simulink model "PNEUMA"  (R2023b)
settings: Solver=ode23tb  StartTime=0  StopTime=3600  FixedStep=0.001  MaxStep=time_step_new  RelTol=0.01  EnableMultiTasking=on
values from neighbouring files (symbols this model uses):
  A = 20.9    [Gas_Exchange_IC.m]    (also in getPneumonia.m = (LF1-LF2)/(1-exp(Rresolve*(t2(end)-t2(1)))))
  a1 = 0.3836    [Dissociation_Spencer_IC.m]    (also in Gas_Exchange_IC.m; Respiratory_IC.m)
  a2 = 1.819    [Dissociation_Spencer_IC.m]    (also in Gas_Exchange_IC.m; Respiratory_IC.m)
  alpha1 = 0.02598    [Dissociation_Spencer_IC.m]    (also in Gas_Exchange_IC.m; Respiratory_IC.m)
  alpha2 = 0.05591    [Dissociation_Spencer_IC.m]    (also in Gas_Exchange_IC.m; Respiratory_IC.m)
  B = 92.8    [Gas_Exchange_IC.m]    (also in getPneumonia.m = LungFunction(end)-A)
  beta1 = 0.012275    [Dissociation_Spencer_IC.m]    (also in Gas_Exchange_IC.m; Respiratory_IC.m)
  beta2 = 0.03255    [Dissociation_Spencer_IC.m]    (also in Gas_Exchange_IC.m; Respiratory_IC.m)
  C = 10570    [Gas_Exchange_IC.m]
  C1 = 9    [Dissociation_Spencer_IC.m]    (also in Gas_Exchange_IC.m; Respiratory_IC.m)
  C2 = 87.00    (= 87)    [Dissociation_Spencer_IC.m]    (also in Gas_Exchange_IC.m; Respiratory_IC.m)
  Circadian_Period = 24    [Respiratory_IC.m]    (also in State_UA_Khoo_IC.m)
  CvCO2IC = 0.5116    [Body_Khoo_IC.m]    (also in Gas_Exchange_IC.m; Respiratory_IC.m = 0.5247)
  CvO2IC = 0.1672    [Body_Khoo_IC.m]    (also in Gas_Exchange_IC.m; Respiratory_IC.m = 0.1639)
  D = -5.251    [Gas_Exchange_IC.m]
  Dead1CO2IC = 0.1020    (= 0.102)    [Dead_Space_Khoo_IC.m]    (also in Gas_Exchange_IC.m; Respiratory_IC.m = 39.5616)
  Dead1O2IC = 149.8824    [Dead_Space_Khoo_IC.m]    (also in Gas_Exchange_IC.m; Respiratory_IC.m = 104.3637)
  Dead2CO2IC = 0.5274    [Dead_Space_Khoo_IC.m]    (also in Gas_Exchange_IC.m; Respiratory_IC.m = 39.6736)
  Dead2O2IC = 149.3923    [Dead_Space_Khoo_IC.m]    (also in Gas_Exchange_IC.m; Respiratory_IC.m = 104.2258)
  Dead3CO2IC = 2.2996    [Dead_Space_Khoo_IC.m]    (also in Gas_Exchange_IC.m; Respiratory_IC.m = 39.8127)
  Dead3O2IC = 147.3503    [Dead_Space_Khoo_IC.m]    (also in Gas_Exchange_IC.m; Respiratory_IC.m = 104.0505)
  Dead4CO2IC = 8.2293    [Dead_Space_Khoo_IC.m]    (also in Gas_Exchange_IC.m; Respiratory_IC.m = 40.0061)
  Dead4O2IC = 140.5179    [Dead_Space_Khoo_IC.m]    (also in Gas_Exchange_IC.m; Respiratory_IC.m = 103.8005)
  Dead5CO2IC = 22.0757    [Dead_Space_Khoo_IC.m]    (also in Gas_Exchange_IC.m; Respiratory_IC.m = 40.3359)
  Dead5O2IC = 124.5641    [Dead_Space_Khoo_IC.m]    (also in Gas_Exchange_IC.m; Respiratory_IC.m = 103.3579)
  DtotalIC = 0.3    [NeuroMuscular_IC.m]    (also in Respiratory_IC.m = 0.32)
  E_CW = 5    [Pleural_Schuessler_IC.m]    (also in Pmus_Flow_Younes_IC.m; Resp_Mech_IC.m; Respiratory_IC.m)
  E_L = 5    [Pleural_Schuessler_IC.m]    (also in Pmus_Flow_Younes_IC.m; Resp_Mech_IC.m; Respiratory_IC.m)
  fc = 0.4/60    (= 0.00666666666667)    [Respiratory_IC.m]    (also in State_UA_Khoo_IC.m)
  fcs_max = 47.78    [Cardiovascular_IC.m]    (also in Reflex_Ursino_IC.m)
  fcs_min = 2.52    [Cardiovascular_IC.m]    (also in Reflex_Ursino_IC.m)
  fcs_zero = 25    [Respiratory_IC.m]
  FlowIC = 0    [Pmus_Flow_Younes_IC.m]    (also in Resp_Mech_IC.m; Respiratory_IC.m)
  fp_inf = 6.3    [Respiratory_IC.m]
  fp_zero = 3.2    [Respiratory_IC.m]
  fs_inf = 2.10    (= 2.1)    [Respiratory_IC.m]
  fs_zero = 16.11    [Respiratory_IC.m]
  ftbs_min = 0.1    [Cardiovascular_IC.m]    (also in SA_Node_Ursino_IC.m)
  gc = 0.008/60    (= 0.000133333333333)    [Respiratory_IC.m]    (also in State_UA_Khoo_IC.m)
  h = 0.0183    [Brain_Khoo_IC.m]    (also in Gas_Exchange_IC.m; Respiratory_IC.m)
  HP_basal = 0.58    [Cardiovascular_IC.m]    (also in SA_Node_Ursino_IC.m)
  Ic = 45    [Gas_Exchange_IC.m]    (also in Respiratory_IC.m; Vent_Drive_Khoo_IC.m)
  IpCO2 = 38    [Gas_Exchange_IC.m]    (also in Respiratory_IC.m; Vent_Drive_Khoo_IC.m)
  IpO2 = 102.4    [Gas_Exchange_IC.m]    (also in Respiratory_IC.m; Vent_Drive_Khoo_IC.m)
  K1 = 13    [Dissociation_Spencer_IC.m]    (also in Gas_Exchange_IC.m; Respiratory_IC.m)
  K2 = 194.4    [Dissociation_Spencer_IC.m]    (also in Gas_Exchange_IC.m; Respiratory_IC.m)
  k_cs = 11.758    [Cardiovascular_IC.m]    (also in Reflex_Ursino_IC.m)
  k_p = 7.06    [Respiratory_IC.m]
  k_s = 0.07    [Respiratory_IC.m]
  lambda = 863    [Gas_Exchange_IC.m]    (also in Lungs_Khoo_IC.m; Respiratory_IC.m)
  Mech_Vent_pressure = 17    [Mech_vent_test.m]
  MRbCO2 = 0.0517    [Brain_Khoo_IC.m]    (also in Gas_Exchange_IC.m; Respiratory_IC.m)
  MRCO2 = 0.0033    [Body_Khoo_IC.m]    (also in Gas_Exchange_IC.m; Respiratory_IC.m)
  MRO2 = 0.0038    [Body_Khoo_IC.m]    (also in Gas_Exchange_IC.m; Respiratory_IC.m)
  NM_block_gain = 1    [Mech_vent_test.m]
  PACO2_delayIC = 39.6041    [Cardio_Mix_Lange_IC.m]    (also in Gas_Exchange_IC.m; Respiratory_IC.m = 40.4448)
  PaCO2firstIC = 0.2150    (= 0.215)    [Cardio_Mix_Lange_IC.m]    (also in Gas_Exchange_IC.m; Respiratory_IC.m = -0.2465)
  PACO2IC = 37.1484    [Gas_Exchange_IC.m]    (also in Lungs_Khoo_IC.m; Respiratory_IC.m = 40.9432)
  PaCO2secondIC = 38.4577    [Cardio_Mix_Lange_IC.m]    (also in Gas_Exchange_IC.m; Respiratory_IC.m = 40.3928)
  PAO2_delayIC = 103.8436    [Cardio_Mix_Lange_IC.m]    (also in Gas_Exchange_IC.m; Respiratory_IC.m = 103.1223)
  PaO2firstIC = -0.2838    [Cardio_Mix_Lange_IC.m]    (also in Gas_Exchange_IC.m; Respiratory_IC.m = 0.3557)
  PAO2IC = 107.1983    [Gas_Exchange_IC.m]    (also in Lungs_Khoo_IC.m; Respiratory_IC.m = 102.5153)
  PaO2secondIC = 105.4828    [Cardio_Mix_Lange_IC.m]    (also in Gas_Exchange_IC.m; Respiratory_IC.m = 103.1435)
  PbCO2IC = 48.2858    [Brain_Khoo_IC.m]    (also in Gas_Exchange_IC.m; Respiratory_IC.m = 48.5383)
  PICO2 = 0    [Dead_Space_Khoo_IC.m]    (also in Gas_Exchange_IC.m; Respiratory_IC.m)
  PIO2 = 150    [Dead_Space_Khoo_IC.m]    (also in Gas_Exchange_IC.m; Respiratory_IC.m)
  PIO2_change = -90    [Mech_vent_test.m]    (also in Respiratory_IC.m = 0)
  Pn = 90    [Cardiovascular_IC.m]    (also in Reflex_Ursino_IC.m)
  Pt_frcIC1 = 0    [Pmus_Flow_Younes_IC.m]    (also in Resp_Mech_IC.m; Respiratory_IC.m)
  Pt_frcIC2 = 0    [Pmus_Flow_Younes_IC.m]    (also in Resp_Mech_IC.m; Respiratory_IC.m)
  QdBo = 0.8333    [Brain_Khoo_IC.m]    (also in Gas_Exchange_IC.m; Respiratory_IC.m)
  R_AW = 1.27    [Pleural_Schuessler_IC.m]    (also in Pmus_Flow_Younes_IC.m; Resp_Mech_IC.m; Respiratory_IC.m)
  R_CW = 1.03    [Pleural_Schuessler_IC.m]    (also in Pmus_Flow_Younes_IC.m; Resp_Mech_IC.m; Respiratory_IC.m)
  R_L = 1.69    [Pleural_Schuessler_IC.m]    (also in Pmus_Flow_Younes_IC.m; Resp_Mech_IC.m; Respiratory_IC.m)
  RC = 0.06    [Pleural_Schuessler_IC.m]    (also in Pmus_Flow_Younes_IC.m; Resp_Mech_IC.m; Respiratory_IC.m)
  rc = 0.2/60    (= 0.00333333333333)    [Respiratory_IC.m]    (also in State_UA_Khoo_IC.m)
  SbCO2 = 0.3600    (= 0.36)    [Brain_Khoo_IC.m]    (also in Gas_Exchange_IC.m; Respiratory_IC.m)
  SCO2 = 0.0043    [Brain_Khoo_IC.m]    (also in Gas_Exchange_IC.m; Respiratory_IC.m)
  SWAo = 0.007    [Respiratory_IC.m]    (also in State_UA_Khoo_IC.m)
  T1 = 1    [Cardio_Mix_Lange_IC.m]    (also in Gas_Exchange_IC.m; Respiratory_IC.m)
  T2 = 2    [Cardio_Mix_Lange_IC.m]    (also in Gas_Exchange_IC.m; Respiratory_IC.m)
  t_end_new = 4*24*60*60    (= 345600)    [Mech_vent_test.m]
  t_end_UA = 0    [Respiratory_IC.m]    (also in State_UA_Khoo_IC.m)
  t_Mech_Vent_duration = 0    [Mech_vent_test.m]
  t_Mech_Vent_start = 0    [Mech_vent_test.m]
  t_Mueller_duration = 0    [NeuroMuscular_IC.m]
  t_Mueller_insp = 0    [NeuroMuscular_IC.m]
  t_Mueller_start = 0    [NeuroMuscular_IC.m]
  t_NM_block_duration = 0    [Mech_vent_test.m]
  t_NM_block_start = 0    [Mech_vent_test.m]
  t_O2_duration = 0    [Mech_vent_test.m]    (also in Respiratory_IC.m)
  t_O2_start = 0    [Mech_vent_test.m]    (also in Respiratory_IC.m)
  t_start_new = 0    [Mech_vent_test.m]
  t_start_UA = 0    [Respiratory_IC.m]    (also in State_UA_Khoo_IC.m)
  t_valsalva_duration = 0    [NeuroMuscular_IC.m]
  t_valsalva_insp = 0    [NeuroMuscular_IC.m]
  t_valsalva_start = 0    [NeuroMuscular_IC.m]
  time_step = time_step    [acquire_data.m]    (also in acquire_data_save.m)
  VC = 5    [Pmus_Flow_Younes_IC.m]    (also in Resp_Mech_IC.m; Respiratory_IC.m)
  Vdead1 = 0.03    [Dead_Space_Khoo_IC.m]    (also in Gas_Exchange_IC.m; Respiratory_IC.m)
  Vdead2 = 0.03    [Dead_Space_Khoo_IC.m]    (also in Gas_Exchange_IC.m; Respiratory_IC.m)
  Vdead3 = 0.03    [Dead_Space_Khoo_IC.m]    (also in Gas_Exchange_IC.m; Respiratory_IC.m)
  Vdead4 = 0.03    [Dead_Space_Khoo_IC.m]    (also in Gas_Exchange_IC.m; Respiratory_IC.m)
  Vdead5 = 0.03    [Dead_Space_Khoo_IC.m]    (also in Gas_Exchange_IC.m; Respiratory_IC.m)
  Ventilator_rate = 12    [Mech_vent_test.m]
  VTCO2 = 15    [Body_Khoo_IC.m]    (also in Gas_Exchange_IC.m; Respiratory_IC.m)
  VtIC = 0    [Pmus_Flow_Younes_IC.m]    (also in Resp_Mech_IC.m; Respiratory_IC.m)
  VTO2 = 6    [Body_Khoo_IC.m]    (also in Gas_Exchange_IC.m; Respiratory_IC.m)
  Z = 0.0227    [Dissociation_Spencer_IC.m]    (also in Gas_Exchange_IC.m; Respiratory_IC.m)
undefined symbols (not defined in the file or in its folder): A_0_ua, alpha_E_FFA_Heart, alpha_E_FFA_muscle, alpha_E_GLC_Heart, alpha_E_GLC_muscle, alpha_E_GLY_muscle, alpha_E_PYR_muscle, alpha_E_TGL_adipose, alpha_E_TGL_GI, alpha_E_TGL_Heart, alpha_E_TGL_muscle, Arousal_UAIC, C_ua_awake, Cbp, Cbv, Ce_0, Cep, Cev, Chp, Chv, Cla, Clamp_class, Cmp, Cmv, Cpa, CPAP_pressure, Cpp, Cpv, Cra, Csa, Csp, Csv, CvbO2_n, CvhO2_n, CvmO2_n, DAY, delay, DietBlock, Dx, Fb, fchemo_max, fchemo_min, fchemoIC, flsIC, Ftas_I0, ftas_min, ftas_r0, FVC_activation, gain_E, Gamma, Gas_sleep, Gas_sleepM, Gb, Gblock, GbO2, Gbs_sleep, gcc_sa, gcc_sb, gcc_sp, Gclamp ... (+144)
libraries: simulink x4, dspstat3 x4, simulink_extras x2
(part 6 of 8)

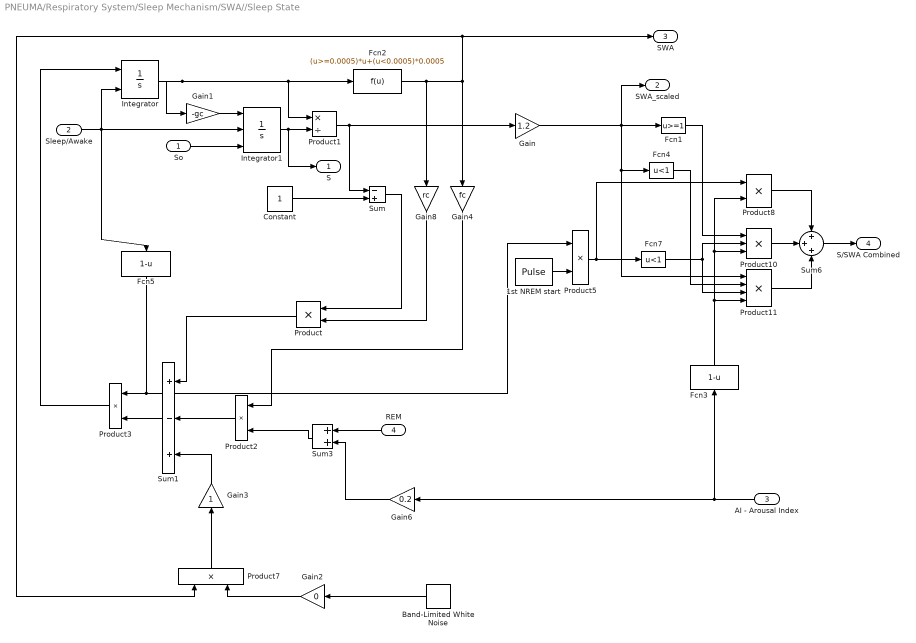
== system PNEUMA/Respiratory System/Sleep Mechanism/SWA//Sleep State ==
  So : Inport
  Sleep/Awake : Inport  Port=2
  AI - Arousal Index : Inport  Port=3
  REM : Inport  Port=4
  1st NREM start : DiscretePulseGenerator  PulseType=Time based  Period=Circadian_Period*3600  PulseWidth=100 - 85 *1.8 /Circadian_Period  PhaseDelay=3600*1.8*0.85+5
  Band-Limited White Noise : simulink/Sources/Band-Limited White Noise  Cov=[0.1]  Ts=0.1  seed=[23341]
  Constant : Constant
  Fcn1 : Fcn  Expr=u>=1
  Fcn2 : Fcn  Expr=(u>=0.0005)*u+(u<0.0005)*0.0005
  Fcn3 : Fcn  Expr=1-u
  Fcn4 : Fcn  Expr=u<1
  Fcn5 : Fcn  Expr=1-u
  Fcn7 : Fcn  Expr=u<1
  Gain : Gain  Gain=1.2
  Gain1 : Gain  Gain=-gc  SaturateOnIntegerOverflow=on  OutDataTypeStr=Inherit: Same as input  ParamDataTypeStr=Inherit: Same as input
  Gain2 : Gain  Gain=0  SaturateOnIntegerOverflow=on  OutDataTypeStr=Inherit: Same as input  ParamDataTypeStr=Inherit: Same as input
  Gain3 : Gain  SaturateOnIntegerOverflow=on  OutDataTypeStr=Inherit: Same as input  ParamDataTypeStr=Inherit: Same as input
  Gain4 : Gain  Gain=fc  SaturateOnIntegerOverflow=on  OutDataTypeStr=Inherit: Same as input  ParamDataTypeStr=Inherit: Same as input
  Gain6 : Gain  Gain=0.2  SaturateOnIntegerOverflow=on  OutDataTypeStr=Inherit: Same as input  ParamDataTypeStr=Inherit: Same as input
  Gain8 : Gain  Gain=rc  SaturateOnIntegerOverflow=on  OutDataTypeStr=Inherit: Same as input  ParamDataTypeStr=Inherit: Same as input
  Integrator : Integrator  ExternalReset=either  InitialCondition=SWAo  LimitOutput=on  UpperSaturationLimit=1  LowerSaturationLimit=0
  Integrator1 : Integrator  ExternalReset=falling  InitialConditionSource=external  InitialCondition=0.8  LimitOutput=on
  Product{,2..3,7..8} (5 alike) : Product  InputSameDT=on  SaturateOnIntegerOverflow=on  OutDataTypeStr=Inherit: Same as first input
  Product1 : Product  Inputs=*/  InputSameDT=on  SaturateOnIntegerOverflow=on  OutDataTypeStr=Inherit: Same as first input
  Product10 : Product  Inputs=3  InputSameDT=on  SaturateOnIntegerOverflow=on  OutDataTypeStr=Inherit: Same as first input
  Product11 : Product  Inputs=4  InputSameDT=on  SaturateOnIntegerOverflow=on  OutDataTypeStr=Inherit: Same as first input
  Product5 : Product  Inputs=**  InputSameDT=on  SaturateOnIntegerOverflow=on  OutDataTypeStr=Inherit: Same as first input
  Sum : Sum  Inputs=-+  InputSameDT=on  SaturateOnIntegerOverflow=on  OutDataTypeStr=Inherit: Same as first input
  Sum1 : Sum  Inputs=+-+  InputSameDT=on  SaturateOnIntegerOverflow=on  OutDataTypeStr=Inherit: Same as first input
  Sum3 : Sum  InputSameDT=on  SaturateOnIntegerOverflow=on  OutDataTypeStr=Inherit: Same as first input
  Sum6 : Sum  Inputs=+++  InputSameDT=on  SaturateOnIntegerOverflow=on  OutDataTypeStr=Inherit: Same as first input
  S : Outport
  SWA_scaled : Outport  Port=2
  SWA : Outport  Port=3
  S/SWA Combined : Outport  Port=4
  wires:
  Fcn4/1 -> Product11/2
  Fcn7/1 -> Product11/3, Product10/2
  Product10/1 -> Sum6/2
  Product11/1 -> Sum6/3
  Sum6/1 -> S/SWA Combined/1
  Product8/1 -> Sum6/1
  Gain2/1 -> Product7/2
  Product7/1 -> Gain3/1
  Gain6/1 -> Sum3/2
  AI - Arousal Index/1 -> Gain6/1, Fcn3/1
  Sum3/1 -> Product2/2
  Constant/1 -> Sum/2
  Product1/1 -> Sum/1, Gain/1
  Gain1/1 -> Integrator1/1
  Integrator/1 -> Product1/1, Fcn2/1, Gain1/1
  Sum/1 -> Product/1
  Product/1 -> Sum1/1
  Product2/1 -> Sum1/2
  Gain3/1 -> Sum1/3
  Integrator1/1 -> Product1/2, S/1
  Sleep/Awake/1 -> Integrator1/2, Fcn5/1, Integrator/2
  So/1 -> Integrator1/3
  Fcn2/1 -> Gain4/1, Product7/1, SWA/1, Gain8/1
  Gain/1 -> SWA_scaled/1, Fcn1/1, Product11/1, Fcn4/1
  Gain4/1 -> Product2/1
  Gain8/1 -> Product/2
  Sum1/1 -> Product3/2
  Product3/1 -> Integrator/1
  Fcn5/1 -> Product3/1, Product5/1
  Fcn3/1 -> Product8/2, Product10/3, Product11/4
  Band-Limited White Noise/1 -> Gain2/1
  Product5/1 -> Fcn7/1, Product8/1
  1st NREM start/1 -> Product5/2
  Fcn1/1 -> Product10/1
  REM/1 -> Sum3/1

== system PNEUMA/Respiratory System/Sleep Mechanism/Saving CircadianProcess ==
  In1 : Inport
  Clock : Clock
  Gain : Gain  Gain=1/(3600*24*DAY)
  Rounding Function : Rounding
  Switch Case : SwitchCase  CaseConditions={0,1,2,3,4,5,6,7,8}  SampleTime=sampletime
  Switch Case Action Subsystem : Subsystem  TreatAsAtomicUnit=on
  Switch Case Action Subsystem1 : Subsystem  TreatAsAtomicUnit=on
  Switch Case Action Subsystem2 : Subsystem  TreatAsAtomicUnit=on
  Switch Case Action Subsystem3 : Subsystem  TreatAsAtomicUnit=on
  Switch Case Action Subsystem4 : Subsystem  TreatAsAtomicUnit=on
  Switch Case Action Subsystem5 : Subsystem  TreatAsAtomicUnit=on
  Switch Case Action Subsystem6 : Subsystem  TreatAsAtomicUnit=on
  Switch Case Action Subsystem7 : Subsystem  TreatAsAtomicUnit=on
  Switch Case Action Subsystem8 : Subsystem  TreatAsAtomicUnit=on
  Switch Case Action Subsystem9 : Subsystem  TreatAsAtomicUnit=on
  wires:
  Clock/1 -> Gain/1
  Switch Case/1 -> Switch Case Action Subsystem/Action
  Switch Case/2 -> Switch Case Action Subsystem1/Action
  Switch Case/3 -> Switch Case Action Subsystem2/Action
  Switch Case/10 -> Switch Case Action Subsystem3/Action
  Rounding Function/1 -> Switch Case/1
  In1/1 -> Switch Case Action Subsystem/1(In1), Switch Case Action Subsystem1/1(In1), Switch Case Action Subsystem2/1(In1), Switch Case Action Subsystem5/1(In1), Switch Case Action Subsystem3/1(In1), Switch Case Action Subsystem9/1(In1), Switch Case Action Subsystem8/1(In1), Switch Case Action Subsystem7/1(In1), Switch Case Action Subsystem6/1(In1), Switch Case Action Subsystem4/1(In1)
  Gain/1 -> Rounding Function/1
  Switch Case/4 -> Switch Case Action Subsystem4/Action
  Switch Case/5 -> Switch Case Action Subsystem5/Action
  Switch Case/6 -> Switch Case Action Subsystem6/Action
  Switch Case/7 -> Switch Case Action Subsystem7/Action
  Switch Case/8 -> Switch Case Action Subsystem8/Action
  Switch Case/9 -> Switch Case Action Subsystem9/Action

== system PNEUMA/Respiratory System/Sleep Mechanism/Triggered Subsystem ==
  In1 : Inport
  Trigger : TriggerPort  VariantControl=(inherit)
  Out1 : Outport
  wires:
  In1/1 -> Out1/1

== system PNEUMA/Respiratory System/Upper_Airway_Mechanism/State-dependent Upper Airway model ==
  SI Sleep Wake State Index : Inport
  AI - Arousal Index : Inport  Port=2
  External Pressure : Inport  Port=3
  Sleep/Awake : Inport  Port=4
  SWA/S : Inport  Port=5
  Airway Cond Saturation2 : Saturate  UpperLimit=1  LowerLimit=0
  Fcn1 : Fcn  Expr="((u(1) >=1.0) * u(2) * (1 + 0.3 * (1 - u(3)) * (1-u(4)) )  + ( u(1)<1.0) * u(1) * u(2) ) *(1- u(5))* u(1)"
  Integrator : Integrator  ExternalReset=rising  InitialCondition=Arousal_UAIC
  Mux1 : Mux  Inputs=5
  PE gain2 : Gain  Gain=1/15  SaturateOnIntegerOverflow=on  OutDataTypeStr=Inherit: Same as input  ParamDataTypeStr=Inherit: Same as input
  S_UA : Constant  Value=0.05
  sum3 : Sum  Inputs=-+  InputSameDT=on  SaturateOnIntegerOverflow=on  OutDataTypeStr=Inherit: Same as first input
  tag scope: Arousal_UAIC=global
  wires:
  AI - Arousal Index/1 -> Integrator/2, Mux1/5
  SI Sleep Wake State Index/1 -> Mux1/1
  SWA/S/1 -> Mux1/3
  Sleep/Awake/1 -> Mux1/4
  S_UA/1 -> sum3/2
  sum3/1 -> Airway Cond Saturation2/1
  External Pressure/1 -> PE gain2/1
  PE gain2/1 -> sum3/1
  Mux1/1 -> Fcn1/1
  Airway Cond Saturation2/1 -> Mux1/2
  Fcn1/1 -> Integrator/1
  Integrator/1 -> [Arousal_UAIC]

== system PNEUMA/Respiratory System/Upper_Airway_Mechanism/Upper_Airway_Model ==
  SI Sleep Wake State Index : Inport
  Respiratory Rhythm : Inport  Port=2
  Q_total Total Respiratory Flow Airways : Inport  Port=3
  Pleural Pressure : Inport  Port=4
  Tidal Volume : Inport  Port=5
  Total Ventilatory Drive : Inport  Port=6
  Sleep/awake : Inport  Port=7
  Enable : EnablePort
  " Flow in Upper Airway" : Subsystem
  " Pressure in Upper Airway" : Subsystem
  Coefficient1 : Gain  SaturateOnIntegerOverflow=on  OutDataTypeStr=Inherit: Same as input  ParamDataTypeStr=Inherit: Same as input
  Mux : Mux  Inputs=2
  Sum2 : Sum  SaturateOnIntegerOverflow=on
  Upper Airway Conductance3 : Subsystem
  Upper Airway Scope : Scope  NumInputPorts=12
  Upper_Airway_Compliance : Subsystem
  "Y_ua Upper Airway Conductance " : Outport  InitialOutput=[0]
  wires:
  Q_total Total Respiratory Flow Airways/1 -> Upper Airway Scope/8, Coefficient1/1  "Q_total"
  SI Sleep Wake State Index/1 -> Upper_Airway_Compliance/1("SI Sleep Wake State Index "), Upper Airway Scope/1  "SI Sleep Wake State Index"
  Pleural Pressure/1 -> Upper Airway Scope/4, " Pressure in Upper Airway"/1(P_pl Pleural Pressure)  "P_pl Pleural Pressure"
  Sum2/1 -> " Pressure in Upper Airway"/2(Q_la Lower Airway Flow), Upper Airway Scope/10  "Q_la Lower Airway Flow"
  " Pressure in Upper Airway"/1("P_ua Upper Airway Pressure ") -> " Flow in Upper Airway"/2(P_ua Pressure in Upper Airways), Upper Airway Conductance3/2(P_ua_Upper Airway Pressure), Mux/2, Upper Airway Scope/5  "P_ua"
  Upper Airway Conductance3/2(P_crit) -> Mux/1  "P_crit"
  Upper_Airway_Compliance/1(C_ua Upper Airway Compliance) -> " Flow in Upper Airway"/1(C_ua Upper Airway Compliance), Upper Airway Conductance3/1(C_ua_Upper_Airway_Compliance), Upper Airway Scope/11  "C_ua Upper Airway Copmliance"
  " Flow in Upper Airway"/1("Q_ua Upper Airway Flow ") -> Upper Airway Scope/9, Sum2/1  "Q_ua Upper Airway Flow"
  Upper Airway Conductance3/1(Y_ua_Upper Airway Conductance) -> Upper Airway Scope/12, "Y_ua Upper Airway Conductance "/1  "Y_ua Upper Airway Conductance"
  Total Ventilatory Drive/1 -> Upper Airway Scope/2  "Ventilatory Drive"
  Mux/1 -> Upper Airway Scope/6  "P_ua vs. P_cirt"
  Tidal Volume/1 -> Upper Airway Scope/7  "Tidal Volume"
  Respiratory Rhythm/1 -> Upper Airway Scope/3  "Respiratory Rhythm"
  Sleep/awake/1 -> Upper_Airway_Compliance/2(Sleep/awake)
  Coefficient1/1 -> Sum2/2

== system PNEUMA/Ventilator/Saving CONTROLLER/Switch Case Action Subsystem ==
  In1 : Inport
  Action Port : ActionPort  ActionPortLabel=case [ 0 ]:
  To File : ToFile  Filename=CONTROLLER1.mat  MatrixName=CONTROLLER  SampleTime=sampletime
  wires:
  In1/1 -> To File/1

== system PNEUMA/Ventilator/Saving CONTROLLER/Switch Case Action Subsystem1 ==
  In1 : Inport
  Action Port : ActionPort  ActionPortLabel=case [ 1 ]:
  To File : ToFile  Filename=CONTROLLER2.mat  MatrixName=CONTROLLER  SampleTime=sampletime
  wires:
  In1/1 -> To File/1

== system PNEUMA/Ventilator/Saving CONTROLLER/Switch Case Action Subsystem2 ==
  In1 : Inport
  Action Port : ActionPort  ActionPortLabel=case [ 2 ]:
  To File : ToFile  Filename=CONTROLLER3.mat  MatrixName=CONTROLLER  SampleTime=sampletime
  wires:
  In1/1 -> To File/1

== system PNEUMA/Ventilator/Saving CONTROLLER/Switch Case Action Subsystem3 ==
  In1 : Inport
  Action Port : ActionPort  ActionPortLabel=default:
  To File : ToFile  Filename=CONTROLLER10.mat  MatrixName=CONTROLLER  SampleTime=sampletime
  wires:
  In1/1 -> To File/1

== system PNEUMA/Ventilator/Saving CONTROLLER/Switch Case Action Subsystem4 ==
  In1 : Inport
  Action Port : ActionPort  ActionPortLabel=case [ 3 ]:
  To File : ToFile  Filename=CONTROLLER4.mat  MatrixName=CONTROLLER  SampleTime=sampletime
  wires:
  In1/1 -> To File/1

== system PNEUMA/Ventilator/Saving CONTROLLER/Switch Case Action Subsystem5 ==
  In1 : Inport
  Action Port : ActionPort  ActionPortLabel=case [ 4 ]:
  To File : ToFile  Filename=CONTROLLER5.mat  MatrixName=CONTROLLER  SampleTime=sampletime
  wires:
  In1/1 -> To File/1

== system PNEUMA/Ventilator/Saving CONTROLLER/Switch Case Action Subsystem6 ==
  In1 : Inport
  Action Port : ActionPort  ActionPortLabel=case [ 5 ]:
  To File : ToFile  Filename=CONTROLLER6.mat  MatrixName=CONTROLLER  SampleTime=sampletime
  wires:
  In1/1 -> To File/1

== system PNEUMA/Ventilator/Saving CONTROLLER/Switch Case Action Subsystem7 ==
  In1 : Inport
  Action Port : ActionPort  ActionPortLabel=case [ 6 ]:
  To File : ToFile  Filename=CONTROLLER7.mat  MatrixName=CONTROLLER  SampleTime=sampletime
  wires:
  In1/1 -> To File/1

== system PNEUMA/Ventilator/Saving CONTROLLER/Switch Case Action Subsystem8 ==
  In1 : Inport
  Action Port : ActionPort  ActionPortLabel=case [ 7 ]:
  To File : ToFile  Filename=CONTROLLER8.mat  MatrixName=CONTROLLER  SampleTime=sampletime
  wires:
  In1/1 -> To File/1

== system PNEUMA/Ventilator/Saving CONTROLLER/Switch Case Action Subsystem9 ==
  In1 : Inport
  Action Port : ActionPort  ActionPortLabel=case [ 8 ]:
  To File : ToFile  Filename=CONTROLLER9.mat  MatrixName=CONTROLLER  SampleTime=sampletime
  wires:
  In1/1 -> To File/1

== system PNEUMA/Ventilator/Ventilator Controller/Inspiratory O2 Partial Pressure ==
  Step : Step  Time=begin_time  Before=init_value  After=final_value  SampleTime=0
  Step1 : Step  Time=end_time  After=init_value-final_value  SampleTime=0
  Sum : Sum  Inputs=|++  InputSameDT=on  SaturateOnIntegerOverflow=on  OutDataTypeStr=Inherit: Same as first input
  Out1 : Outport
  wires:
  Sum/1 -> Out1/1
  Step1/1 -> Sum/2
  Step/1 -> Sum/1

== system PNEUMA/Ventilator/Ventilator Controller/Mean Arterial Pressure Estimation ==
  note: known discrete sample time
  ABP : Inport
  Gain : Gain  Gain=1/3
  Moving Maximum : dspstat3/Moving Maximum  SpecifyWindowLength=on  WindowLength=50  SimulateUsing=Code generation
  Moving Minimum : dspstat3/Moving Minimum  SpecifyWindowLength=on  WindowLength=50  SimulateUsing=Code generation
  Rate Transition : RateTransition  OutPortSampleTime=0.2
  Sum : Sum  Inputs=+|+
  Sum1 : Sum  Inputs=|+-
  MAP : Outport
  wires:
  ABP/1 -> Rate Transition/1  "ABP"
  Sum1/1 -> Gain/1  "PulseP"
  Moving Minimum/1 -> Sum/2, Sum1/2  "DiastolicP"
  Sum/1 -> MAP/1  "MAP"
  Moving Maximum/1 -> Sum1/1  "SystolicP"
  Gain/1 -> Sum/1
  Rate Transition/1 -> Moving Maximum/1, Moving Minimum/1

== system PNEUMA/Ventilator/Ventilator Controller/Mech Vent Pressure ==
  Step : Step  Time=begin_time  Before=init_value  After=final_value  SampleTime=0
  Step1 : Step  Time=end_time  After=init_value-final_value  SampleTime=0
  Sum : Sum  Inputs=|++  InputSameDT=on  SaturateOnIntegerOverflow=on  OutDataTypeStr=Inherit: Same as first input
  Out1 : Outport
  wires:
  Step/1 -> Sum/1
  Step1/1 -> Sum/2
  Sum/1 -> Out1/1

== system PNEUMA/Ventilator/Ventilator Controller/NM Block gain ==
  Step : Step  Time=begin_time  Before=1  After=NM_block_gain  SampleTime=0
  Step1 : Step  Time=end_time  After=1-NM_block_gain  SampleTime=0
  Sum : Sum  Inputs=+-  InputSameDT=on  SaturateOnIntegerOverflow=on  OutDataTypeStr=Inherit: Same as first input
  Out1 : Outport
  wires:
  Step/1 -> Sum/1
  Step1/1 -> Sum/2
  Sum/1 -> Out1/1

== system PNEUMA/Ventilator/Ventilator Controller/Peak Breath CO2 Detector ==
  BCO2 : Inport
  Moving Maximum : dspstat3/Moving Maximum  SpecifyWindowLength=on  WindowLength=50  SimulateUsing=Code generation
  Rate Transition : RateTransition  OutPortSampleTime=0.2
  peakBCO2 : Outport
  wires:
  Moving Maximum/1 -> peakBCO2/1  "peakBCO2"
  BCO2/1 -> Rate Transition/1
  Rate Transition/1 -> Moving Maximum/1

== system PNEUMA/Ventilator/Ventilator Controller/Peak Tidal Volume Detector ==
  Vt : Inport
  Moving Maximum : dspstat3/Moving Maximum  SpecifyWindowLength=on  WindowLength=50  SimulateUsing=Code generation
  Rate Transition : RateTransition  OutPortSampleTime=0.2
  peakVt : Outport
  wires:
  Moving Maximum/1 -> peakVt/1  "peakVt"
  Vt/1 -> Rate Transition/1
  Rate Transition/1 -> Moving Maximum/1

== system PNEUMA/Ventilator/Ventilator Controller/Ventilator rate ==
  Step : Step  Time=begin_time  After=Ventilator_rate  SampleTime=0
  Step1 : Step  Time=end_time  After=Ventilator_rate  SampleTime=0
  Sum : Sum  Inputs=+-  InputSameDT=on  SaturateOnIntegerOverflow=on  OutDataTypeStr=Inherit: Same as first input
  Out1 : Outport
  wires:
  Step/1 -> Sum/1
  Step1/1 -> Sum/2
  Sum/1 -> Out1/1

== system PNEUMA/Cardiovascular System/Left Heart/Saving PVleft/Switch Case Action Subsystem ==
  In1 : Inport
  Action Port : ActionPort  ActionPortLabel=case [ 0 ]:
  To File : ToFile  Filename=PVleft1.mat  MatrixName=PLeft_VLeft  SampleTime=0.1
  wires:
  In1/1 -> To File/1

== system PNEUMA/Cardiovascular System/Left Heart/Saving PVleft/Switch Case Action Subsystem1 ==
  In1 : Inport
  Action Port : ActionPort  ActionPortLabel=case [ 1 ]:
  To File : ToFile  Filename=PVleft2.mat  MatrixName=PLeft_VLeft  SampleTime=0.1
  wires:
  In1/1 -> To File/1

== system PNEUMA/Cardiovascular System/Left Heart/Saving PVleft/Switch Case Action Subsystem2 ==
  In1 : Inport
  Action Port : ActionPort  ActionPortLabel=case [ 2 ]:
  To File : ToFile  Filename=PVleft3.mat  MatrixName=PLeft_VLeft  SampleTime=0.1
  wires:
  In1/1 -> To File/1

== system PNEUMA/Cardiovascular System/Left Heart/Saving PVleft/Switch Case Action Subsystem3 ==
  In1 : Inport
  Action Port : ActionPort  ActionPortLabel=default:
  To File : ToFile  Filename=PVleft10.mat  MatrixName=PLeft_VLeft  SampleTime=0.1
  wires:
  In1/1 -> To File/1

== system PNEUMA/Cardiovascular System/Left Heart/Saving PVleft/Switch Case Action Subsystem4 ==
  In1 : Inport
  Action Port : ActionPort  ActionPortLabel=case [ 3 ]:
  To File : ToFile  Filename=PVleft4.mat  MatrixName=PLeft_VLeft  SampleTime=0.1
  wires:
  In1/1 -> To File/1

== system PNEUMA/Cardiovascular System/Left Heart/Saving PVleft/Switch Case Action Subsystem5 ==
  In1 : Inport
  Action Port : ActionPort  ActionPortLabel=case [ 4 ]:
  To File : ToFile  Filename=PVleft5.mat  MatrixName=PLeft_VLeft  SampleTime=0.1
  wires:
  In1/1 -> To File/1

== system PNEUMA/Cardiovascular System/Left Heart/Saving PVleft/Switch Case Action Subsystem6 ==
  In1 : Inport
  Action Port : ActionPort  ActionPortLabel=case [ 5 ]:
  To File : ToFile  Filename=PVleft6.mat  MatrixName=PLeft_VLeft  SampleTime=0.1
  wires:
  In1/1 -> To File/1

== system PNEUMA/Cardiovascular System/Left Heart/Saving PVleft/Switch Case Action Subsystem7 ==
  In1 : Inport
  Action Port : ActionPort  ActionPortLabel=case [ 6 ]:
  To File : ToFile  Filename=PVleft7.mat  MatrixName=PLeft_VLeft  SampleTime=0.1
  wires:
  In1/1 -> To File/1

== system PNEUMA/Cardiovascular System/Left Heart/Saving PVleft/Switch Case Action Subsystem8 ==
  In1 : Inport
  Action Port : ActionPort  ActionPortLabel=case [ 7 ]:
  To File : ToFile  Filename=PVleft8.mat  MatrixName=PLeft_VLeft  SampleTime=0.1
  wires:
  In1/1 -> To File/1

== system PNEUMA/Cardiovascular System/Left Heart/Saving PVleft/Switch Case Action Subsystem9 ==
  In1 : Inport
  Action Port : ActionPort  ActionPortLabel=case [ 8 ]:
  To File : ToFile  Filename=PVleft9.mat  MatrixName=PLeft_VLeft  SampleTime=0.1
  wires:
  In1/1 -> To File/1

== system PNEUMA/Cardiovascular System/Local Flow Regulation/Cerebral Circulation Regulation/Subsystem ==
  QbpIC : Inport
  If : If  IfExpression=u1 == 0  ShowElse=off
  If Action Subsystem : Subsystem  TreatAsAtomicUnit=on
  Step 10sec : Step  Time=0  After=5  SampleTime=0
  Step1 : Step  Time=5  After=-5  SampleTime=0
  Sum : Sum  Inputs=|++
  Sum1 : Sum  Inputs=|++
  Qbp : Outport
  wires:
  Step 10sec/1 -> Sum/1
  Step1/1 -> Sum/2
  Sum/1 -> Sum1/2, If/1
  If/1 -> If Action Subsystem/Action
  QbpIC/1 -> If Action Subsystem/1(In1)
  Sum1/1 -> Qbp/1
  If Action Subsystem/1(Out1) -> Sum1/1

== system PNEUMA/Cardiovascular System/Local Flow Regulation/Coronary Circulation Regulation2/Subsystem ==
  Q : Inport
  If : If  IfExpression=u1 == 0  ShowElse=off
  If Action Subsystem : Subsystem  TreatAsAtomicUnit=on
  Step 10sec : Step  Time=0  SampleTime=0
  Step1 : Step  After=-1  SampleTime=0
  Sum : Sum  Inputs=|++
  Sum1 : Sum  Inputs=|++
  Qhp : Outport
  wires:
  Step 10sec/1 -> Sum/1
  Step1/1 -> Sum/2
  Sum/1 -> Sum1/2, If/1
  If/1 -> If Action Subsystem/Action
  Q/1 -> If Action Subsystem/1(In1)
  Sum1/1 -> Qhp/1
  If Action Subsystem/1(Out1) -> Sum1/1

== system PNEUMA/Cardiovascular System/Local Flow Regulation/Muscular Circulation Regulation1/Subsystem ==
  Q : Inport
  If : If  IfExpression=u1 == 0  ShowElse=off
  If Action Subsystem : Subsystem  TreatAsAtomicUnit=on
  Step 10sec : Step  Time=0  After=5  SampleTime=0
  Step1 : Step  After=-5  SampleTime=0
  Sum : Sum  Inputs=|++
  Sum1 : Sum  Inputs=|++
  Qmp : Outport
  wires:
  Step 10sec/1 -> Sum/1
  Step1/1 -> Sum/2
  Sum/1 -> Sum1/2, If/1
  If/1 -> If Action Subsystem/Action
  Q/1 -> If Action Subsystem/1(In1)
  Sum1/1 -> Qmp/1
  If Action Subsystem/1(Out1) -> Sum1/1

== system PNEUMA/Cardiovascular System/SA-node and Autonomic Control/Left Ventricle/SubSystem1 ==
  _ : Inport
  + : Inport  Port=2
  Saturation : Saturate  UpperLimit=10000  LowerLimit=0
  Sum : Sum  Inputs=|-+  InputSameDT=on  SaturateOnIntegerOverflow=on  OutDataTypeStr=Inherit: Same as first input
  Out : Outport
  wires:
  _/1 -> Sum/1
  +/1 -> Sum/2
  Sum/1 -> Saturation/1
  Saturation/1 -> Out/1

== system PNEUMA/Cardiovascular System/SA-node and Autonomic Control/RR Interval/If Action Subsystem ==
  In1 : Inport
  Action Port : ActionPort  ActionPortLabel=if(u1 <0)
  Out1 : Outport
  wires:
  In1/1 -> Out1/1

== system PNEUMA/Cardiovascular System/SA-node and Autonomic Control/RR Interval/Saving varHeartPeriod ==
  In1 : Inport
  Clock : Clock
  Gain : Gain  Gain=1/(3600*24*7)
  Rounding Function : Rounding
  Switch Case : SwitchCase  CaseConditions={0,1,2,3,4,5,6,7,8}  SampleTime=0.1
  Switch Case Action Subsystem : Subsystem  TreatAsAtomicUnit=on
  Switch Case Action Subsystem1 : Subsystem  TreatAsAtomicUnit=on
  Switch Case Action Subsystem2 : Subsystem  TreatAsAtomicUnit=on
  Switch Case Action Subsystem3 : Subsystem  TreatAsAtomicUnit=on
  Switch Case Action Subsystem4 : Subsystem  TreatAsAtomicUnit=on
  Switch Case Action Subsystem5 : Subsystem  TreatAsAtomicUnit=on
  Switch Case Action Subsystem6 : Subsystem  TreatAsAtomicUnit=on
  Switch Case Action Subsystem7 : Subsystem  TreatAsAtomicUnit=on
  Switch Case Action Subsystem8 : Subsystem  TreatAsAtomicUnit=on
  Switch Case Action Subsystem9 : Subsystem  TreatAsAtomicUnit=on
  wires:
  Clock/1 -> Gain/1
  Switch Case/1 -> Switch Case Action Subsystem/Action
  Switch Case/2 -> Switch Case Action Subsystem1/Action
  Switch Case/3 -> Switch Case Action Subsystem2/Action
  Switch Case/10 -> Switch Case Action Subsystem3/Action
  Rounding Function/1 -> Switch Case/1
  In1/1 -> Switch Case Action Subsystem/1(In1), Switch Case Action Subsystem1/1(In1), Switch Case Action Subsystem2/1(In1), Switch Case Action Subsystem5/1(In1), Switch Case Action Subsystem3/1(In1), Switch Case Action Subsystem9/1(In1), Switch Case Action Subsystem8/1(In1), Switch Case Action Subsystem7/1(In1), Switch Case Action Subsystem6/1(In1), Switch Case Action Subsystem4/1(In1)
  Gain/1 -> Rounding Function/1
  Switch Case/4 -> Switch Case Action Subsystem4/Action
  Switch Case/5 -> Switch Case Action Subsystem5/Action
  Switch Case/6 -> Switch Case Action Subsystem6/Action
  Switch Case/7 -> Switch Case Action Subsystem7/Action
  Switch Case/8 -> Switch Case Action Subsystem8/Action
  Switch Case/9 -> Switch Case Action Subsystem9/Action

== system PNEUMA/Cardiovascular System/SA-node and Autonomic Control/Right Ventricle/SubSystem1 ==
  _ : Inport
  + : Inport  Port=2
  Saturation : Saturate  UpperLimit=10000  LowerLimit=0
  Sum : Sum  Inputs=|-+  InputSameDT=on  SaturateOnIntegerOverflow=on  OutDataTypeStr=Inherit: Same as first input
  Out : Outport
  wires:
  Saturation/1 -> Out/1
  Sum/1 -> Saturation/1
  +/1 -> Sum/2
  _/1 -> Sum/1

== system PNEUMA/Cardiovascular System/SA-node and Autonomic Control/phi/SubSystem ==
  In1 : Inport
  Trigger : TriggerPort  VariantControl=(inherit)
  Data Store Write : DataStoreWrite  IndexOptions=Index vector (dialog)  Indices=1  OutputSizes=1
  wires:
  In1/1 -> Data Store Write/1

== system PNEUMA/Cardiovascular System/Systemic/Systemic Arteries/SubSystem ==
  _ : Inport
  + : Inport  Port=2
  Saturation : Saturate  UpperLimit=10000  LowerLimit=0
  Sum : Sum  Inputs=|-+  InputSameDT=on  SaturateOnIntegerOverflow=on  OutDataTypeStr=Inherit: Same as first input
  Out : Outport
  wires:
  _/1 -> Sum/1
  +/1 -> Sum/2
  Sum/1 -> Saturation/1
  Saturation/1 -> Out/1

== system PNEUMA/Cardiovascular System/Systemic/Systemic Peripheral & Venous Circulation/SubSystem1 ==
  + : Inport
  _ : Inport  Port=2
  Saturation : Saturate  UpperLimit=10000  LowerLimit=0
  Sum : Sum  Inputs=|+-  InputSameDT=on  SaturateOnIntegerOverflow=on  OutDataTypeStr=Inherit: Same as first input
  Out : Outport
  wires:
  Saturation/1 -> Out/1
  Sum/1 -> Saturation/1
  _/1 -> Sum/2
  +/1 -> Sum/1

== system PNEUMA/Cardiovascular System/Systemic/Systemic Peripheral & Venous Circulation/SubSystem2 ==
  _1 : Inport
  _2 : Inport  Port=2
  _3 : Inport  Port=3
  _4 : Inport  Port=4
  _5 : Inport  Port=5
  + : Inport  Port=6
  Saturation : Saturate  UpperLimit=10000  LowerLimit=0  ZeroCross=off
  Sum : Sum  Inputs=|-----+  InputSameDT=on  SaturateOnIntegerOverflow=on  OutDataTypeStr=Inherit: Same as first input
  Out : Outport
  wires:
  Saturation/1 -> Out/1
  Sum/1 -> Saturation/1
  _1/1 -> Sum/1
  _2/1 -> Sum/2
  _3/1 -> Sum/3
  _4/1 -> Sum/4
  _5/1 -> Sum/5
  +/1 -> Sum/6

== system PNEUMA/Cardiovascular System/Systemic/Systemic Peripheral & Venous Circulation/SubSystem3 ==
  + : Inport
  _ : Inport  Port=2
  Saturation : Saturate  UpperLimit=10000  LowerLimit=0
  Sum : Sum  Inputs=|+-  InputSameDT=on  SaturateOnIntegerOverflow=on  OutDataTypeStr=Inherit: Same as first input
  Out : Outport
  wires:
  Saturation/1 -> Out/1
  Sum/1 -> Saturation/1
  _/1 -> Sum/2
  +/1 -> Sum/1

== system PNEUMA/Cardiovascular System/Systemic/Systemic Peripheral & Venous Circulation/SubSystem4 ==
  + : Inport
  _ : Inport  Port=2
  Saturation : Saturate  UpperLimit=10000  LowerLimit=0
  Sum : Sum  Inputs=|+-  InputSameDT=on  SaturateOnIntegerOverflow=on  OutDataTypeStr=Inherit: Same as first input
  Out : Outport
  wires:
  Saturation/1 -> Out/1
  Sum/1 -> Saturation/1
  _/1 -> Sum/2
  +/1 -> Sum/1

== system PNEUMA/Cardiovascular System/Systemic/Systemic Peripheral & Venous Circulation/SubSystem5 ==
  + : Inport
  _ : Inport  Port=2
  Saturation : Saturate  UpperLimit=10000  LowerLimit=0
  Sum : Sum  Inputs=|+-  InputSameDT=on  SaturateOnIntegerOverflow=on  OutDataTypeStr=Inherit: Same as first input
  Out : Outport
  wires:
  Saturation/1 -> Out/1
  Sum/1 -> Saturation/1
  _/1 -> Sum/2
  +/1 -> Sum/1

== system PNEUMA/Cardiovascular System/Systemic/Vena Cava/SubSystem3 ==
  + : Inport
  _ : Inport  Port=2
  Saturation : Saturate  UpperLimit=10000  LowerLimit=0
  Sum : Sum  Inputs=|+-  InputSameDT=on  SaturateOnIntegerOverflow=on  OutDataTypeStr=Inherit: Same as first input
  Out : Outport
  wires:
  Saturation/1 -> Out/1
  Sum/1 -> Saturation/1
  _/1 -> Sum/2
  +/1 -> Sum/1

== system PNEUMA/Cardiovascular System/TPR Change/Saving TPR/Switch Case Action Subsystem ==
  In1 : Inport
  Action Port : ActionPort  ActionPortLabel=case [ 0 ]:
  To File : ToFile  Filename=TPR1.mat  MatrixName=TPR  SampleTime=0.1
  wires:
  In1/1 -> To File/1

== system PNEUMA/Cardiovascular System/TPR Change/Saving TPR/Switch Case Action Subsystem1 ==
  In1 : Inport
  Action Port : ActionPort  ActionPortLabel=case [ 1 ]:
  To File : ToFile  Filename=TPR2.mat  MatrixName=TPR  SampleTime=0.1
  wires:
  In1/1 -> To File/1

== system PNEUMA/Cardiovascular System/TPR Change/Saving TPR/Switch Case Action Subsystem2 ==
  In1 : Inport
  Action Port : ActionPort  ActionPortLabel=case [ 2 ]:
  To File : ToFile  Filename=TPR3.mat  MatrixName=TPR  SampleTime=0.1
  wires:
  In1/1 -> To File/1

== system PNEUMA/Cardiovascular System/TPR Change/Saving TPR/Switch Case Action Subsystem3 ==
  In1 : Inport
  Action Port : ActionPort  ActionPortLabel=default:
  To File : ToFile  Filename=TPR10.mat  MatrixName=TPR  SampleTime=0.1
  wires:
  In1/1 -> To File/1

== system PNEUMA/Cardiovascular System/TPR Change/Saving TPR/Switch Case Action Subsystem4 ==
  In1 : Inport
  Action Port : ActionPort  ActionPortLabel=case [ 3 ]:
  To File : ToFile  Filename=TPR4.mat  MatrixName=TPR  SampleTime=0.1
  wires:
  In1/1 -> To File/1

== system PNEUMA/Cardiovascular System/TPR Change/Saving TPR/Switch Case Action Subsystem5 ==
  In1 : Inport
  Action Port : ActionPort  ActionPortLabel=case [ 4 ]:
  To File : ToFile  Filename=TPR5.mat  MatrixName=TPR  SampleTime=0.1
  wires:
  In1/1 -> To File/1

== system PNEUMA/Cardiovascular System/TPR Change/Saving TPR/Switch Case Action Subsystem6 ==
  In1 : Inport
  Action Port : ActionPort  ActionPortLabel=case [ 5 ]:
  To File : ToFile  Filename=TPR6.mat  MatrixName=TPR  SampleTime=0.1
  wires:
  In1/1 -> To File/1

== system PNEUMA/Cardiovascular System/TPR Change/Saving TPR/Switch Case Action Subsystem7 ==
  In1 : Inport
  Action Port : ActionPort  ActionPortLabel=case [ 6 ]:
  To File : ToFile  Filename=TPR7.mat  MatrixName=TPR  SampleTime=0.1
  wires:
  In1/1 -> To File/1

== system PNEUMA/Cardiovascular System/TPR Change/Saving TPR/Switch Case Action Subsystem8 ==
  In1 : Inport
  Action Port : ActionPort  ActionPortLabel=case [ 7 ]:
  To File : ToFile  Filename=TPR8.mat  MatrixName=TPR  SampleTime=0.1
  wires:
  In1/1 -> To File/1

== system PNEUMA/Cardiovascular System/TPR Change/Saving TPR/Switch Case Action Subsystem9 ==
  In1 : Inport
  Action Port : ActionPort  ActionPortLabel=case [ 8 ]:
  To File : ToFile  Filename=TPR9.mat  MatrixName=TPR  SampleTime=0.1
  wires:
  In1/1 -> To File/1

== system PNEUMA/Central Neural Control/VARIABLE RESPIRATORY RHYTHM1/Variable Breathing Period Reset/If Action Subsystem ==
  In1 : Inport
  Action Port : ActionPort  ActionPortLabel=if(u1 <0)
  Out1 : Outport
  wires:
  In1/1 -> Out1/1

== system PNEUMA/Central Neural Control/VARIABLE RESPIRATORY RHYTHM1/Variable Breathing Period Reset/Saving BreathingPeriod ==
  In1 : Inport
  Clock : Clock
  Gain : Gain  Gain=1/(3600*24*DAY)
  Rounding Function : Rounding
  Switch Case : SwitchCase  CaseConditions={0,1,2,3,4,5,6,7,8}  SampleTime=sampletime
  Switch Case Action Subsystem : Subsystem  TreatAsAtomicUnit=on
  Switch Case Action Subsystem1 : Subsystem  TreatAsAtomicUnit=on
  Switch Case Action Subsystem2 : Subsystem  TreatAsAtomicUnit=on
  Switch Case Action Subsystem3 : Subsystem  TreatAsAtomicUnit=on
  Switch Case Action Subsystem4 : Subsystem  TreatAsAtomicUnit=on
  Switch Case Action Subsystem5 : Subsystem  TreatAsAtomicUnit=on
  Switch Case Action Subsystem6 : Subsystem  TreatAsAtomicUnit=on
  Switch Case Action Subsystem7 : Subsystem  TreatAsAtomicUnit=on
  Switch Case Action Subsystem8 : Subsystem  TreatAsAtomicUnit=on
  Switch Case Action Subsystem9 : Subsystem  TreatAsAtomicUnit=on
  wires:
  Clock/1 -> Gain/1
  Switch Case/1 -> Switch Case Action Subsystem/Action
  Switch Case/2 -> Switch Case Action Subsystem1/Action
  Switch Case/3 -> Switch Case Action Subsystem2/Action
  Switch Case/10 -> Switch Case Action Subsystem3/Action
  Rounding Function/1 -> Switch Case/1
  In1/1 -> Switch Case Action Subsystem/1(In1), Switch Case Action Subsystem1/1(In1), Switch Case Action Subsystem2/1(In1), Switch Case Action Subsystem4/1(In1), Switch Case Action Subsystem5/1(In1), Switch Case Action Subsystem3/1(In1), Switch Case Action Subsystem9/1(In1), Switch Case Action Subsystem8/1(In1), Switch Case Action Subsystem7/1(In1), Switch Case Action Subsystem6/1(In1)
  Gain/1 -> Rounding Function/1
  Switch Case/4 -> Switch Case Action Subsystem4/Action
  Switch Case/5 -> Switch Case Action Subsystem5/Action
  Switch Case/6 -> Switch Case Action Subsystem6/Action
  Switch Case/7 -> Switch Case Action Subsystem7/Action
  Switch Case/8 -> Switch Case Action Subsystem8/Action
  Switch Case/9 -> Switch Case Action Subsystem9/Action

== system PNEUMA/Central Neural Control/VENTILATORY DRIVE (chemical)/Dynamic Drive/Saving stpres ==
  In1 : Inport
  Clock : Clock
  Gain : Gain  Gain=1/(3600*24*DAY)
  Rounding Function : Rounding
  Switch Case : SwitchCase  CaseConditions={0,1,2,3,4,5,6,7,8}  SampleTime=sampletime
  Switch Case Action Subsystem : Subsystem  TreatAsAtomicUnit=on
  Switch Case Action Subsystem1 : Subsystem  TreatAsAtomicUnit=on
  Switch Case Action Subsystem2 : Subsystem  TreatAsAtomicUnit=on
  Switch Case Action Subsystem3 : Subsystem  TreatAsAtomicUnit=on
  Switch Case Action Subsystem4 : Subsystem  TreatAsAtomicUnit=on
  Switch Case Action Subsystem5 : Subsystem  TreatAsAtomicUnit=on
  Switch Case Action Subsystem6 : Subsystem  TreatAsAtomicUnit=on
  Switch Case Action Subsystem7 : Subsystem  TreatAsAtomicUnit=on
  Switch Case Action Subsystem8 : Subsystem  TreatAsAtomicUnit=on
  Switch Case Action Subsystem9 : Subsystem  TreatAsAtomicUnit=on
  wires:
  Clock/1 -> Gain/1
  Switch Case/1 -> Switch Case Action Subsystem/Action
  Switch Case/2 -> Switch Case Action Subsystem1/Action
  Switch Case/3 -> Switch Case Action Subsystem2/Action
  Switch Case/10 -> Switch Case Action Subsystem3/Action
  Rounding Function/1 -> Switch Case/1
  In1/1 -> Switch Case Action Subsystem/1(In1), Switch Case Action Subsystem1/1(In1), Switch Case Action Subsystem2/1(In1), Switch Case Action Subsystem5/1(In1), Switch Case Action Subsystem3/1(In1), Switch Case Action Subsystem9/1(In1), Switch Case Action Subsystem8/1(In1), Switch Case Action Subsystem7/1(In1), Switch Case Action Subsystem6/1(In1), Switch Case Action Subsystem4/1(In1)
  Gain/1 -> Rounding Function/1
  Switch Case/4 -> Switch Case Action Subsystem4/Action
  Switch Case/5 -> Switch Case Action Subsystem5/Action
  Switch Case/6 -> Switch Case Action Subsystem6/Action
  Switch Case/7 -> Switch Case Action Subsystem7/Action
  Switch Case/8 -> Switch Case Action Subsystem8/Action
  Switch Case/9 -> Switch Case Action Subsystem9/Action

== system PNEUMA/Metabolic Control/Display & Storage/Saving G_I_FFA/Switch Case Action Subsystem ==
  In1 : Inport
  Action Port : ActionPort  ActionPortLabel=case [ 0 ]:
  To File : ToFile  Filename=GIMM_FFA_SEC1.mat  MatrixName=G_I_F_E_Gin_Iin  SampleTime=sampletime*6
  wires:
  In1/1 -> To File/1

== system PNEUMA/Metabolic Control/Display & Storage/Saving G_I_FFA/Switch Case Action Subsystem1 ==
  In1 : Inport
  Action Port : ActionPort  ActionPortLabel=case [ 1 ]:
  To File1 : ToFile  Filename=GIMM_FFA_SEC2.mat  MatrixName=G_I_F_E_Gin_Iin  SampleTime=sampletime*6
  wires:
  In1/1 -> To File1/1

== system PNEUMA/Metabolic Control/Display & Storage/Saving G_I_FFA/Switch Case Action Subsystem2 ==
  In1 : Inport
  Action Port : ActionPort  ActionPortLabel=case [ 2 ]:
  To File : ToFile  Filename=GIMM_FFA_SEC3.mat  MatrixName=G_I_F_E_Gin_Iin  SampleTime=sampletime*6
  wires:
  In1/1 -> To File/1

== system PNEUMA/Metabolic Control/Display & Storage/Saving G_I_FFA/Switch Case Action Subsystem3 ==
  In1 : Inport
  Action Port : ActionPort  ActionPortLabel=default:
  To File : ToFile  Filename=GIMM_FFA_SEC10.mat  MatrixName=G_I_F_E_Gin_Iin  SampleTime=sampletime*6
  wires:
  In1/1 -> To File/1

== system PNEUMA/Metabolic Control/Display & Storage/Saving G_I_FFA/Switch Case Action Subsystem4 ==
  In1 : Inport
  Action Port : ActionPort  ActionPortLabel=case [ 3 ]:
  To File : ToFile  Filename=GIMM_FFA_SEC4.mat  MatrixName=G_I_F_E_Gin_Iin  SampleTime=sampletime*6
  wires:
  In1/1 -> To File/1

== system PNEUMA/Metabolic Control/Display & Storage/Saving G_I_FFA/Switch Case Action Subsystem5 ==
  In1 : Inport
  Action Port : ActionPort  ActionPortLabel=case [ 4 ]:
  To File : ToFile  Filename=GIMM_FFA_SEC5.mat  MatrixName=G_I_F_E_Gin_Iin  SampleTime=sampletime*6
  wires:
  In1/1 -> To File/1

== system PNEUMA/Metabolic Control/Display & Storage/Saving G_I_FFA/Switch Case Action Subsystem6 ==
  In1 : Inport
  Action Port : ActionPort  ActionPortLabel=case [ 5 ]:
  To File : ToFile  Filename=GIMM_FFA_SEC6.mat  MatrixName=G_I_F_E_Gin_Iin  SampleTime=sampletime*6
  wires:
  In1/1 -> To File/1

== system PNEUMA/Metabolic Control/Display & Storage/Saving G_I_FFA/Switch Case Action Subsystem7 ==
  In1 : Inport
  Action Port : ActionPort  ActionPortLabel=case [ 6 ]:
  To File : ToFile  Filename=GIMM_FFA_SEC7.mat  MatrixName=G_I_F_E_Gin_Iin  SampleTime=sampletime*6
  wires:
  In1/1 -> To File/1

== system PNEUMA/Metabolic Control/Display & Storage/Saving G_I_FFA/Switch Case Action Subsystem8 ==
  In1 : Inport
  Action Port : ActionPort  ActionPortLabel=case [ 7 ]:
  To File1 : ToFile  Filename=GIMM_FFA_SEC8.mat  MatrixName=G_I_F_E_Gin_Iin  SampleTime=sampletime*6
  wires:
  In1/1 -> To File1/1

== system PNEUMA/Metabolic Control/Display & Storage/Saving G_I_FFA/Switch Case Action Subsystem9 ==
  In1 : Inport
  Action Port : ActionPort  ActionPortLabel=case [ 8 ]:
  To File1 : ToFile  Filename=GIMM_FFA_SEC9.mat  MatrixName=G_I_F_E_Gin_Iin  SampleTime=sampletime*6
  wires:
  In1/1 -> To File1/1

== system PNEUMA/Metabolic Control/Epinephrine Regulation on Heart and Muscle/Epi Modulation/GI ==
  Ce(t) : Inport
  Fcn3 : Fcn  Expr=u(2) * ( 1+ u(4) * (u(1) - u(3))^2/( u(5)+(u(1) - u(3))^2 ))
  GI: TGL_to_FFA : Constant  Value=[V_0_TGL_GI, Ce_0, lamda_E_TGL_GI, alpha_E_TGL_GI]
  Mux4 : Mux  Inputs=2
  Epi on GI : Outport
  wires:
  Ce(t)/1 -> Mux4/1
  GI: TGL_to_FFA/1 -> Mux4/2
  Mux4/1 -> Fcn3/1
  Fcn3/1 -> Epi on GI/1

== system PNEUMA/Metabolic Control/Epinephrine Regulation on Heart and Muscle/Epi Modulation/GI1 ==
  Ce(t) : Inport
  Fcn3 : Fcn  Expr=u(2) * ( 1+ u(4) * (u(1) - u(3))^2/( u(5)+(u(1) - u(3))^2 ))
  Mux4 : Mux  Inputs=2
  "adipose : TGL_to_FFA" : Constant  Value=[V_0_TGL_adipose, Ce_0, lamda_E_TGL_adipose, alpha_E_TGL_adipose]
  Epi on adipose : Outport
  wires:
  Ce(t)/1 -> Mux4/1
  "adipose : TGL_to_FFA"/1 -> Mux4/2
  Mux4/1 -> Fcn3/1
  Fcn3/1 -> Epi on adipose/1

== system PNEUMA/Metabolic Control/Epinephrine Regulation on Heart and Muscle/Epi Modulation/Heart ==
  Ce(t) : Inport
  Add : Sum  Inputs=++++
  Fcn : Fcn  Expr=u(2) * ( 1+ u(4) * (u(1) - u(3))^2/( u(5)+(u(1) - u(3))^2 ))
  Fcn2 : Fcn  Expr=u(2) * ( 1+ u(4) * (u(1) - u(3))^2/( u(5)+(u(1) - u(3))^2 ))
  Fcn3 : Fcn  Expr=u(2) * ( 1+ u(4) * (u(1) - u(3))^2/( u(5)+(u(1) - u(3))^2 ))
  Heart: FFA_to_ACoA : Constant  Value=[V_0_FFA_Heart, Ce_0, lamda_E_FFA_Heart, alpha_E_FFA_Heart]
  Heart: GLC_to_G6P : Constant  Value=[V_0_GLC_Heart, Ce_0, lamda_E_GLC_Heart, alpha_E_GLC_Heart]
  Heart: GLY_to_G6P : Constant  Value=V_0_GLY_Heart
  Heart: TGL_to_FFA : Constant  Value=[V_0_TGL_Heart, Ce_0, lamda_E_TGL_Heart, alpha_E_TGL_Heart]
  Mux : Mux  Inputs=2
  Mux2 : Mux  Inputs=2
  Mux3 : Mux
  Mux4 : Mux  Inputs=2
  Epi on Heart (Fluxes) : Outport
  Epi on Heart (Sum) : Outport  Port=2
  wires:
  Ce(t)/1 -> Mux/1, Mux2/1, Mux4/1
  Heart: GLC_to_G6P/1 -> Mux/2
  Mux/1 -> Fcn/1
  Heart: GLY_to_G6P/1 -> Mux3/2, Add/2
  Heart: FFA_to_ACoA/1 -> Mux2/2
  Mux2/1 -> Fcn2/1
  Fcn/1 -> Mux3/1, Add/1
  Heart: TGL_to_FFA/1 -> Mux4/2
  Mux4/1 -> Fcn3/1
  Fcn3/1 -> Mux3/4, Add/4
  Fcn2/1 -> Mux3/3, Add/3
  Mux3/1 -> Epi on Heart (Fluxes)/1
  Add/1 -> Epi on Heart (Sum)/1
